simulink model "Regulator"  (R2018b)
settings: Solver=VariableStepAuto  StartTime=0.0  StopTime=10.0  RelTol=1e-3
undefined symbols (not defined in the file): DiscIntNeverNeededParam
libraries: simulink x5
settings Model: Creator=K2  LastModifiedBy=K2

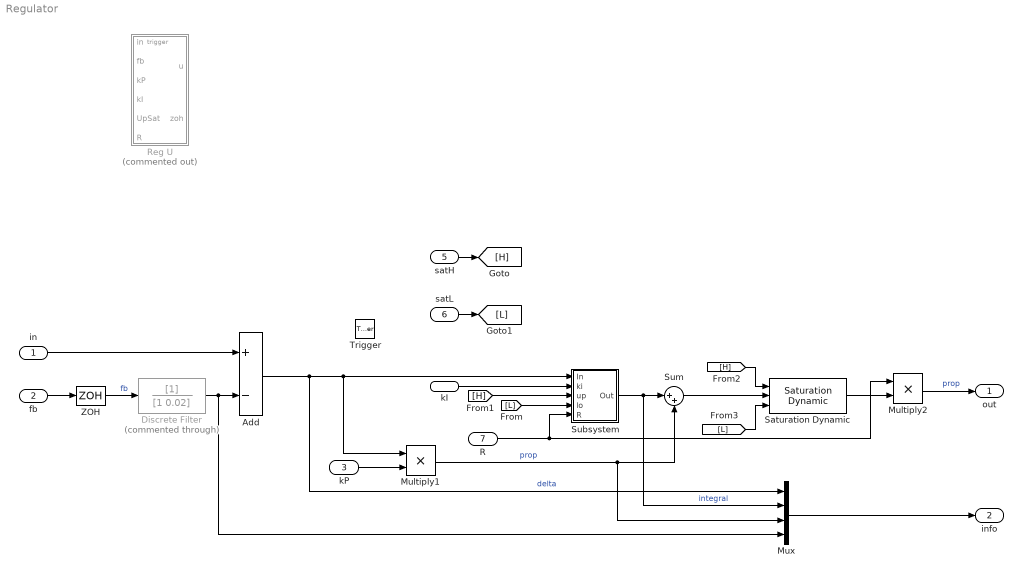
== system Regulator ==
  in : Inport
  fb : Inport  Port=2
  kP : Inport  Port=3
  kI : Inport  Port=4
  satH : Inport  Port=5
  satL : Inport  Port=6
  R : Inport  Port=7
  Trigger : TriggerPort  TriggerType=either  VariantControl=Variant  PortDimensions=1
  Add : Sum  Inputs=+-
  Discrete Filter : DiscreteFilter  Commented=through  Denominator=[1 0.02]
  Multiply1 : Product
  Multiply2 : Product
  Mux : Mux
  Reg U : Subsystem  Commented=on
  Saturation Dynamic : simulink/Discontinuities/Saturation Dynamic  OutMin=[]  OutMax=[]  OutDataTypeStr=Inherit: Same as second input  OutDataType=fixdt(1, 16)  OutScaling=2^-10  DoSatur=off
  Subsystem : Subsystem
  Sum : Sum  Inputs=|++
  ZOH : ZeroOrderHold  SampleTime=-1
  out : Outport  OutDataTypeStr=double
  info : Outport  Port=2
  wires:
  [H] -> Subsystem/3(up)
  Sum/1 -> Saturation Dynamic/2
  [L] -> Subsystem/4(lo)
  Add/1 -> Mux/1, Multiply1/1, Subsystem/1(In)  "delta"
  [L] -> Saturation Dynamic/3
  [H] -> Saturation Dynamic/1
  satL/1 -> [L]
  kI/1 -> Subsystem/2(ki)
  Multiply1/1 -> Mux/3, Sum/2  "prop"
  kP/1 -> Multiply1/2
  satH/1 -> [H]
  in/1 -> Add/1
  Saturation Dynamic/1 -> Multiply2/2
  ZOH/1 -> Discrete Filter/1  "fb"
  fb/1 -> ZOH/1
  R/1 -> Subsystem/5(R), Multiply2/1
  Subsystem/1(Out) -> Mux/2, Sum/1  "integral"
  Mux/1 -> info/1
  Discrete Filter/1 -> Mux/4, Add/2
  Multiply2/1 -> out/1  "prop"

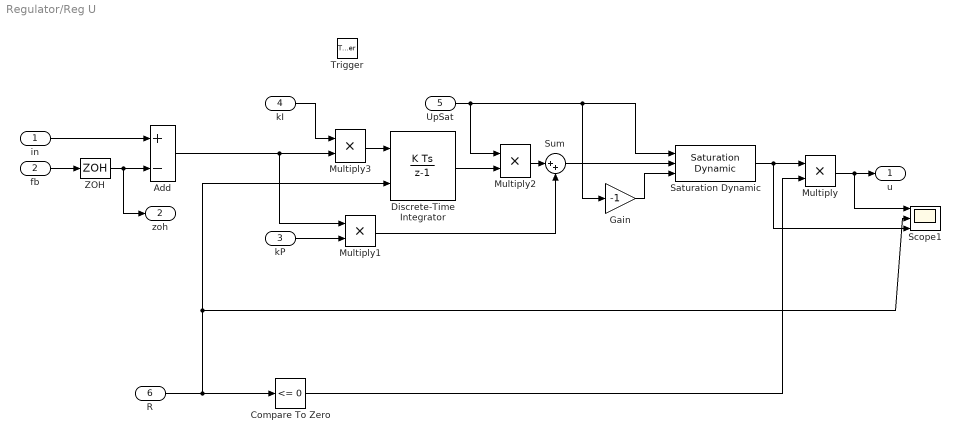
== system Regulator/Reg U ==
  in : Inport
  fb : Inport  Port=2
  kP : Inport  Port=3
  kI : Inport  Port=4
  UpSat : Inport  Port=5
  R : Inport  Port=6
  Trigger : TriggerPort  VariantControl=Variant  PortDimensions=1
  Add : Sum  Inputs=+-
  Compare To Zero : simulink/Logic and Bit Operations/Compare To Zero  relop=<=  OutDataTypeStr=boolean
  Discrete-Time Integrator : DiscreteIntegrator  gainval=1  ExternalReset=level  SampleTime=-1  LimitOutput=on  UpperSaturationLimit=1  LowerSaturationLimit=-1  ICPrevOutput=DiscIntNeverNeededParam  ICPrevScaledInput=DiscIntNeverNeededParam
  Gain : Gain  Gain=-1
  Multiply{,1..3} (4 alike) : Product
  Saturation Dynamic : simulink/Discontinuities/Saturation Dynamic  OutMin=[]  OutMax=[]  OutDataTypeStr=Inherit: Same as second input  OutDataType=fixdt(1, 16)  OutScaling=2^-10  DoSatur=off
  Scope1 : Scope  NumInputPorts=3
  Sum : Sum  Inputs=|++
  ZOH : ZeroOrderHold  SampleTime=-1
  u : Outport
  zoh : Outport  Port=2
  wires:
  fb/1 -> ZOH/1
  in/1 -> Add/1
  Saturation Dynamic/1 -> Scope1/3, Multiply/1
  ZOH/1 -> zoh/1, Add/2
  Multiply/1 -> Scope1/1, u/1
  Compare To Zero/1 -> Multiply/2
  R/1 -> Scope1/2, Discrete-Time Integrator/2, Compare To Zero/1
  Sum/1 -> Saturation Dynamic/2
  kP/1 -> Multiply1/2
  Add/1 -> Multiply1/1, Multiply3/2
  UpSat/1 -> Multiply2/1, Gain/1, Saturation Dynamic/1
  Gain/1 -> Saturation Dynamic/3
  Discrete-Time Integrator/1 -> Multiply2/2
  kI/1 -> Multiply3/1
  Multiply1/1 -> Sum/2
  Multiply2/1 -> Sum/1
  Multiply3/1 -> Discrete-Time Integrator/1

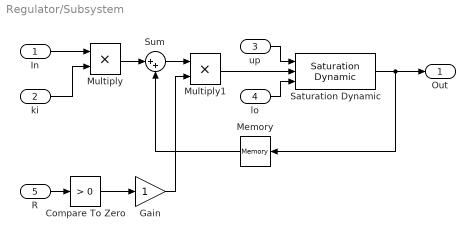
== system Regulator/Subsystem ==
  In : Inport
  ki : Inport  Port=2
  up : Inport  Port=3
  lo : Inport  Port=4
  R : Inport  Port=5
  Compare To Zero : simulink/Logic and Bit Operations/Compare To Zero  relop=>  OutDataTypeStr=boolean
  Gain : Gain  OutDataTypeStr=double
  Memory : Memory  InheritSampleTime=on
  Multiply : Product
  Multiply1 : Product
  Saturation Dynamic : simulink/Discontinuities/Saturation Dynamic  OutMin=[]  OutMax=[]  OutDataTypeStr=Inherit: Same as second input  OutDataType=fixdt(1, 16)  OutScaling=2^-10  DoSatur=off
  Sum : Sum  Inputs=|++
  Out : Outport
  wires:
  In/1 -> Multiply/1
  ki/1 -> Multiply/2
  Multiply/1 -> Sum/1
  Saturation Dynamic/1 -> Out/1, Memory/1
  Multiply1/1 -> Saturation Dynamic/2
  up/1 -> Saturation Dynamic/1
  lo/1 -> Saturation Dynamic/3
  R/1 -> Compare To Zero/1
  Memory/1 -> Sum/2
  Gain/1 -> Multiply1/2
  Compare To Zero/1 -> Gain/1
  Sum/1 -> Multiply1/1
